simulink model "QuarterCarModel"  (R2025a)
settings: Solver=VariableStepAuto  StartTime=0.0  StopTime=15  RelTol=1e-3
undefined symbols (not defined in the file): c1, c2, k1, k2, Kd, Ki, Kp, m1, m2
libraries: slpidlib x1
settings Model: Creator=datnd  LastModifiedBy=datnd

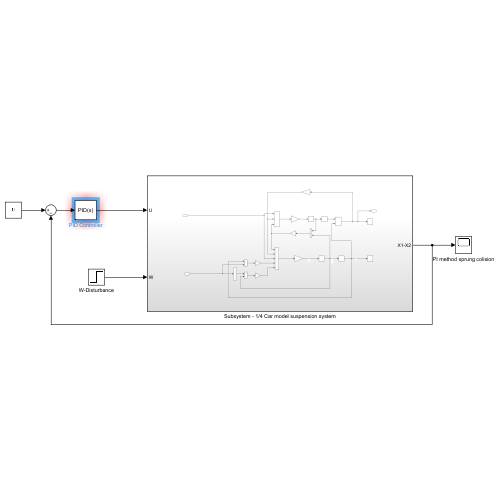
[thumbnail: Simulink's stored preview of the top-level diagram]
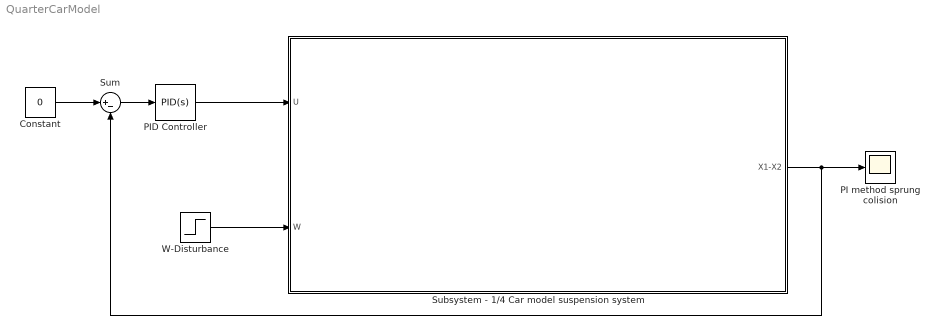
== system QuarterCarModel ==
  Constant : Constant  Value=0
  PI method sprung colision : Scope
      settings: ActiveDisplayYMinimum=-0.075037004787195077  ActiveDisplayYMaximum=0.04157457420216934  DataLoggingVariableName=ScopeData2
  PID Controller : slpidlib/PID Controller  Controller=PID  Form=Parallel  TimeDomain=Continuous-time  UseExternalTs=off  SampleTime=-1  IntegratorMethod=Forward Euler  FilterMethod=Forward Euler  ControllerParametersSource=internal  P=Kp  I=Ki  UseKiTs=off  D=Kd  UseExternalDerivativeSource=off  N=100  UseFilter=on  TunerSelectOption=Transfer Function Based (PID Tuner App)  InitialConditionSource=internal  InitialConditionForIntegrator=0  InitialConditionForFilter=0  DifferentiatorICPrevScaledInput=0  ExternalReset=none  TrackingMode=off  Kt=1  LimitOutput=off  SatLimitsSource=internal  UpperSaturationLimit=inf  LowerSaturationLimit=-inf  LinearizeAsGain=on  AntiWindupMode=none  Kb=1  LimitIntegrator=off  UpperIntegratorSaturationLimit=inf  LowerIntegratorSaturationLimit=-inf  POutMin=[]  POutMax=[]  IOutMin=[]  IOutMax=[]  DOutMin=[]  DOutMax=[]  NOutMin=[]  NOutMax=[]  SumOutMin=[]  SumOutMax=[]  SaturationOutMin=[]  SaturationOutMax=[]  PParamMin=[]  PParamMax=[]  IParamMin=[]  IParamMax=[]  DParamMin=[]  DParamMax=[]  NParamMin=[]  NParamMax=[]  KbParamMin=[]  KbParamMax=[]  KtParamMin=[]  KtParamMax=[]  KbOutMin=[]  KbOutMax=[]  KtOutMin=[]  KtOutMax=[]  IntegratorOutMin=[]  IntegratorOutMax=[]  FilterOutMin=[]  FilterOutMax=[]  SumI1OutMin=[]  SumI1OutMax=[]  SumI2OutMin=[]  SumI2OutMax=[]  SumI3OutMin=[]  SumI3OutMax=[]  SumI4OutMin=[]  SumI4OutMax=[]  SumDOutMin=[]  SumDOutMax=[]  DifferentiatorOutMin=[]  DifferentiatorOutMax=[]  FilterDiffOutCoefMin=[]  FilterDiffOutCoefMax=[]  ReciprocalOutMin=[]  ReciprocalOutMax=[]  SumDenOutMin=[]  SumDenOutMax=[]  SumNumOutMin=[]  SumNumOutMax=[]  DivideOutMin=[]  DivideOutMax=[]  UdiffTsProdOutMin=[]  UdiffTsProdOutMax=[]  NTsProdOutMin=[]  NTsProdOutMax=[]  UintegralTsProdOutMin=[]  UintegralTsProdOutMax=[]  UngainTsProdOutMin=[]  UngainTsProdOutMax=[]  ClampingZeroOutDataTypeStr=Inherit: Inherit via back propagation  ClampingZeroOutMin=[]  ClampingZeroOutMax=[]  FilterDenConstantOutDataTypeStr=Inherit: Inherit via back propagation  FilterDenConstantOutMin=[]  FilterDenConstantOutMax=[]  PCopyOutDataTypeStr=Inherit: Inherit via back propagation  PCopyOutMin=[]  PCopyOutMax=[]  NCopyOutDataTypeStr=Inherit: Inherit via back propagation  NCopyOutMin=[]  NCopyOutMax=[]  IntegratorContinuousStateAttributes=''  IntegratorStateMustResolveToSignalObject=off  IntegratorRTWStateStorageClass=Auto  FilterContinuousStateAttributes=''  FilterStateMustResolveToSignalObject=off  FilterRTWStateStorageClass=Auto  ParallelPVariant=InternalParameters  IdealPVariant=Disabled  IVariant=InternalParameters  DVariant=InternalParameters  IntegratorVariant=Continuous  SatVariant=Disabled  AWVariant=Passthrough  PCopyVariant=Disabled  TRVariant=Disabled  FdbkBlocksVariant=Forward  IdealPFdbkVariant=Disabled  SatFdbkVariant=Disabled  DerivativeFilterVariant=ContFilter  NVariant=InternalParameters  NCopyVariant=Disabled  FilterICVariant=InternalICsFilter  IntegratorICVariant=InternalICs  ExternalResetVariant=Disabled  TRSumVariant=Passthrough  SumFdbkVariant=Disabled  SumVariant=Sum_PID  TsampFilterVariant=InternalTs  TsampNgainVariant=Passthrough  TsampIntegralVariant=Disabled_SignalSpec  ExternalSaturationOutDataTypeStr=Inherit: Same as second input  DerivativeSourceVariant=ErrorSignal  PreIntVariant=InternalPreInt
  Subsystem - 1/4 Car model suspension system : Subsystem
  Sum : Sum  Inputs=|+-
  W-Disturbance : Step  Time=0  After=0.1  SampleTime=1
  wires:
  PID Controller/1 -> Subsystem - 1/4 Car model suspension system/1(U)
  W-Disturbance/1 -> Subsystem - 1/4 Car model suspension system/2(W)
  Subsystem - 1/4 Car model suspension system/1(X1-X2) -> Sum/2, PI method sprung colision/1
  Constant/1 -> Sum/1
  Sum/1 -> PID Controller/1

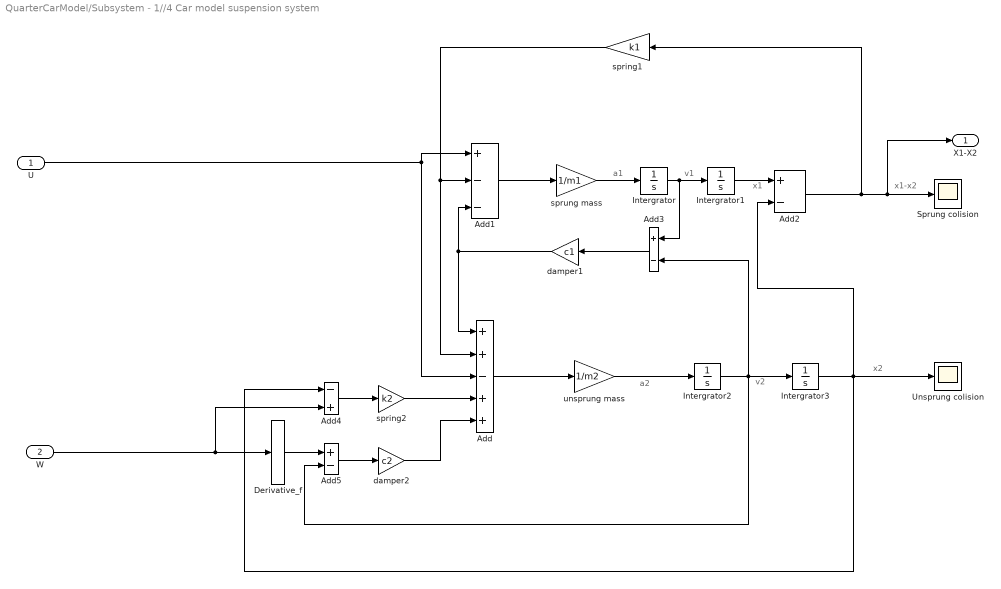
== system QuarterCarModel/Subsystem - 1//4 Car model suspension system ==
  note: a2
  note: v2
  note: v1
  note: x2
  note: x1-x2
  note: x1
  note: a1
  U : Inport
  W : Inport  Port=2
  " spring1" : Gain  Gain=k1
  Add : Sum  Inputs=++-++
  Add1 : Sum  Inputs=+--
  Add2 : Sum  Inputs=+-
  Add3 : Sum  Inputs=+-
  Add4 : Sum  Inputs=-+
  Add5 : Sum  Inputs=+-
  Derivative_f : Derivative
  Intergrator{,1..3} (4 alike) : Integrator
  Sprung colision : Scope
      settings: ActiveDisplayYMinimum=-5.8954508062791371  ActiveDisplayYMaximum=5.1236316864063065
  Unsprung colision : Scope
      settings: ActiveDisplayYMinimum=0.07805042220169453  ActiveDisplayYMaximum=0.11236521240015429
  damper1 : Gain  Gain=c1
  damper2 : Gain  Gain=c2
  spring2 : Gain  Gain=k2
  sprung mass : Gain  Gain=1/m1
  unsprung mass : Gain  Gain=1/m2
  X1-X2 : Outport
  wires:
  sprung mass/1 -> Intergrator/1
  " spring1"/1 -> Add1/2, Add/2
  damper1/1 -> Add1/3, Add/1
  Intergrator3/1 -> Add2/2, Unsprung colision/1, Add4/1
  spring2/1 -> Add/4
  Intergrator1/1 -> Add2/1
  Add1/1 -> sprung mass/1
  Add3/1 -> damper1/1
  Intergrator2/1 -> Add3/2, Add5/2, Intergrator3/1
  U/1 -> Add1/1, Add/3
  Add2/1 -> " spring1"/1, X1-X2/1, Sprung colision/1
  damper2/1 -> Add/5
  W/1 -> Derivative_f/1, Add4/2
  Add5/1 -> damper2/1
  Add/1 -> unsprung mass/1
  Derivative_f/1 -> Add5/1
  unsprung mass/1 -> Intergrator2/1
  Intergrator/1 -> Add3/1, Intergrator1/1
  Add4/1 -> spring2/1
